simulink model "Simulink_spr_4_integratory"  (R2023b)
settings: Solver=VariableStepAuto  StartTime=0.0  StopTime=10.0  RelTol=1e-3
undefined symbols (not defined in the file): c1, c2, k1, k2, m1, m2, x0
settings Model: Creator=Szymon  LastModifiedBy=Szymon

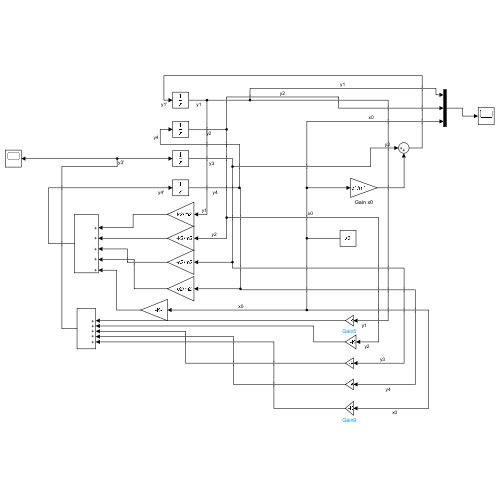
[thumbnail: Simulink's stored preview of the top-level diagram]
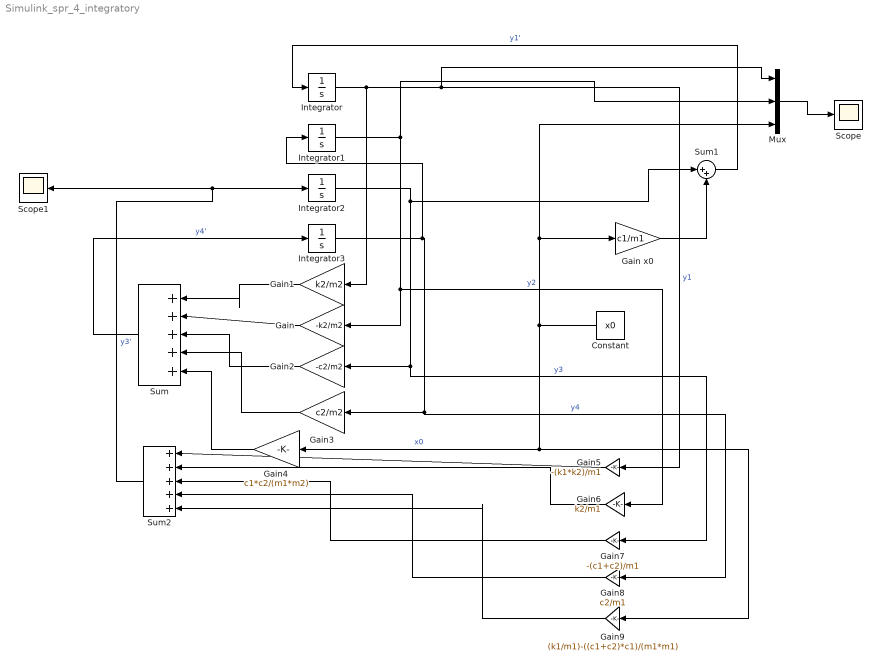
== system Simulink_spr_4_integratory ==
  Constant : Constant  Value=x0
  Gain : Gain  Gain=-k2/m2
  Gain x0 : Gain  Gain=c1/m1
  Gain1 : Gain  Gain=k2/m2
  Gain2 : Gain  Gain=-c2/m2
  Gain3 : Gain  Gain=c2/m2
  Gain4 : Gain  Gain=c1*c2/(m1*m2)
  Gain5 : Gain  Gain=-(k1*k2)/m1
  Gain6 : Gain  Gain=k2/m1
  Gain7 : Gain  Gain=-(c1+c2)/m1
  Gain8 : Gain  Gain=c2/m1
  Gain9 : Gain  Gain=(k1/m1)-((c1+c2)*c1)/(m1*m1)
  Integrator{,1..3} (4 alike) : Integrator
  Mux : Mux  Inputs=3
  Scope : Scope
  Scope1 : Scope
  Sum : Sum  Inputs=|+++++
  Sum1 : Sum  Inputs=|++
  Sum2 : Sum  Inputs=|+++++
  wires:
  Integrator1/1 -> Gain/1, Gain6/1, Mux/2  "y2"
  Sum1/1 -> Integrator/1  "y1'"
  Integrator/1 -> Gain5/1, Mux/1, Gain1/1  "y1"
  Sum2/1 -> Integrator2/1, Scope1/1  "y3'"
  Integrator2/1 -> Gain7/1, Gain2/1, Sum1/1  "y3"
  Sum/1 -> Integrator3/1  "y4'"
  Integrator3/1 -> Integrator1/1, Gain8/1, Gain3/1  "y4"
  Gain1/1 -> Sum/1
  Gain/1 -> Sum/2
  Gain2/1 -> Sum/3
  Gain3/1 -> Sum/4
  Gain4/1 -> Sum/5
  Constant/1 -> Gain9/1, Gain4/1, Gain x0/1, Mux/3  "x0"
  Gain5/1 -> Sum2/1
  Gain8/1 -> Sum2/4
  Gain7/1 -> Sum2/3
  Gain6/1 -> Sum2/2
  Gain9/1 -> Sum2/5
  Gain x0/1 -> Sum1/2
  Mux/1 -> Scope/1
